simulink model "FullControllerPartC"  (R2012b)
settings: Solver=ode45  StartTime=0.0  StopTime=500.0  RelTol=1e-3
settings Model: Creator=Jake  LastModifiedBy=Jake

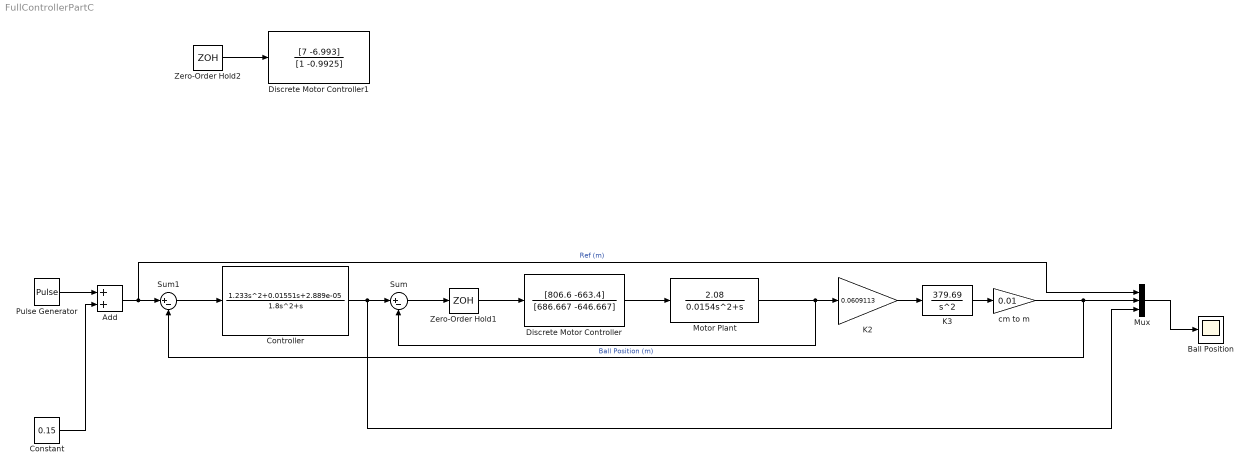
== system FullControllerPartC ==
  Add : Sum
  Ball Position : Scope
      settings: ShowLegends=on  YMin=0  YMax=0.4  MaxDataPoints=350000
  Constant : Constant  Value=0.15
  "Controller " : TransferFcn  Numerator=[1.233 0.01551 2.889e-05]  Denominator=[1.8 1 0]
  Discrete Motor Controller : DiscreteFilter  Numerator=[806.6 -663.4]  Denominator=[686.667 -646.667]
  Discrete Motor Controller1 : DiscreteFilter  Numerator=[7 -6.993]  Denominator=[1 -0.9925]
  "K2 " : Gain  Gain=0.0609113
  K3 : TransferFcn  Numerator=[379.69]  Denominator=[1 0 0]
  Motor Plant : TransferFcn  Numerator=[2.08]  Denominator=[0.0154 1 0]
  Mux : Mux  Inputs=3
  Pulse Generator : DiscretePulseGenerator  PulseType=Time based  Amplitude=0.1  Period=500  PulseWidth=50
  Sum : Sum  Inputs=|+-
  Sum1 : Sum  Inputs=|+-
  Zero-Order Hold1 : ZeroOrderHold  SampleTime=0.003
  Zero-Order Hold2 : ZeroOrderHold  SampleTime=0.003
  cm to m : Gain  Gain=0.01
  wires:
  Motor Plant/1 -> "K2 "/1, Sum/2
  "K2 "/1 -> K3/1
  Zero-Order Hold1/1 -> Discrete Motor Controller/1
  Pulse Generator/1 -> Add/1
  Constant/1 -> Add/2
  Add/1 -> Mux/1, Sum1/1  "Ref (m)"
  Mux/1 -> Ball Position/1
  Discrete Motor Controller/1 -> Motor Plant/1
  Sum/1 -> Zero-Order Hold1/1
  K3/1 -> cm to m/1
  cm to m/1 -> Sum1/2, Mux/2  "Ball Position (m)"
  Zero-Order Hold2/1 -> Discrete Motor Controller1/1
  Sum1/1 -> "Controller "/1
  "Controller "/1 -> Mux/3, Sum/1
